simulink model "sim_pend_free"  (R2023a)
settings: Solver=ode4  StartTime=t0  StopTime=t(end)  FixedStep=h  RelTol=1e-3
values from neighbouring files (symbols this model uses):
  alpha2 = p2(1)    [ident_pend_lsm.m]
  g = 9.81e+00    (= 9.81)    [ident_pend_lsm.m]
  mu2 = p2(2)    [ident_pend_lsm.m]
undefined symbols (not defined in the file or in its folder): phi20
settings Model: Creator=kawata  LastModifiedBy=kawata
settings SolverCC: AlgebraicLoopSolver=TrustRegion
settings DataIOCC: ReturnWorkspaceOutputs=off
settings DebuggingCC: UnconnectedInputMsg=warning  UnconnectedOutputMsg=warning  UnconnectedLineMsg=warning  ArithmeticOperatorsInVariantConditions=warning
settings ModelReferenceCC: EnableRefExpFcnMdlSchedulingChecks=on
settings SFSimCC: SimUseLocalCustomCode=off  CustomCodeUndefinedFunction=UseInterfaceOnly
settings RTWCC: RTWUseLocalCustomCode=off

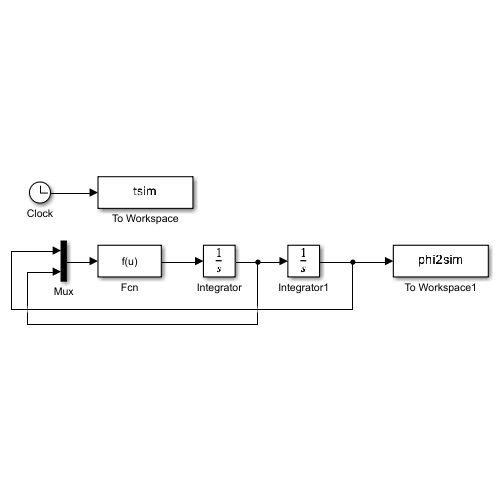
[thumbnail: Simulink's stored preview of the top-level diagram]
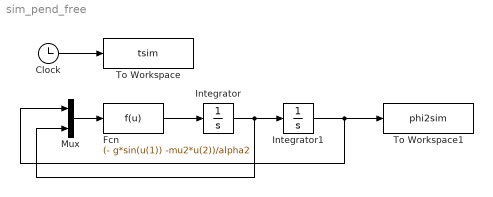
== system sim_pend_free ==
  Clock : Clock
  Fcn : Fcn  Expr=(- g*sin(u(1)) -mu2*u(2))/alpha2
  Integrator : Integrator
  Integrator1 : Integrator  InitialCondition=phi20
  Mux : Mux  Inputs=2
  To Workspace : ToWorkspace  VariableName=tsim  SampleTime=-1
  To Workspace1 : ToWorkspace  VariableName=phi2sim  SampleTime=-1
  wires:
  Mux/1 -> Fcn/1
  Fcn/1 -> Integrator/1
  Integrator/1 -> Mux/2, Integrator1/1
  Integrator1/1 -> To Workspace1/1, Mux/1
  Clock/1 -> To Workspace/1
